simulink model "FuSimple"  (Simulink 5.0)
settings: Solver=ode23tb  StartTime=0.0  StopTime=inf  MaxStep=1/100000  MinStep=1/1000000000  RelTol=1e-6
undefined symbols (not defined in the file or in its folder): get, RFSSimple
libraries: simulink x7, commcontsrc2 x2, dspsnks4 x2
settings Model: LastModifiedBy=efst  SimulationMode=accelerator

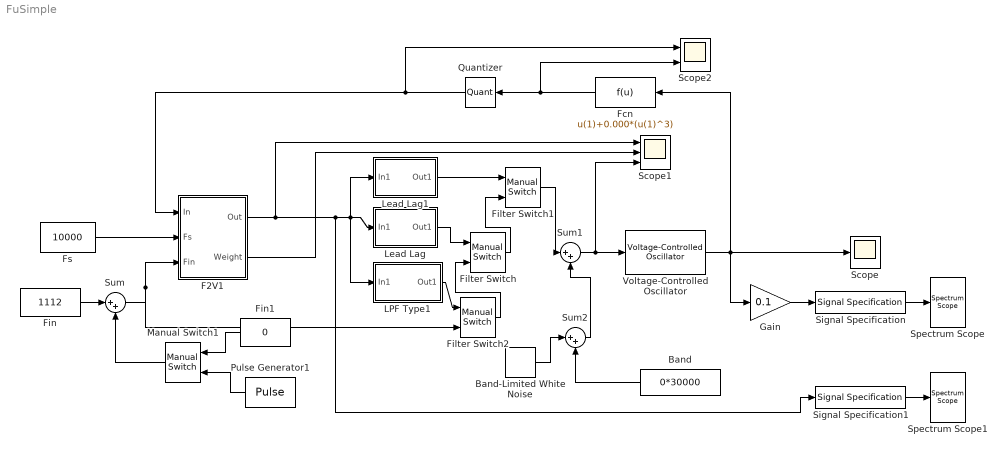
== system FuSimple ==
  Band : Constant  Orientation=left  Value=0*30000
  Band-Limited White Noise : simulink/Sources/Band-Limited White Noise  Cov=[0.0000]  Ts=1/10000  seed=[23341]
  F2V1 : Subsystem
  Fcn : Fcn  Orientation=left  Expr=u(1)+0.000*(u(1)^3)
  Filter Switch : simulink/Signal Routing/Manual Switch  sw=0  action=0
  Filter Switch1 : simulink/Signal Routing/Manual Switch  sw=0  action=0
  Filter Switch2 : simulink/Signal Routing/Manual Switch  sw=0  action=0
  Fin : Constant  Value=1112
  Fin1 : Constant  Orientation=left  Value=0
  Fs : Constant  Value=10000
  Gain : Gain  Gain=0.1  SaturateOnIntegerOverflow=on
  LPF Type1 : Subsystem  TreatAsAtomicUnit=on
  Lead Lag : Subsystem  TreatAsAtomicUnit=on
  Lead Lag1 : Subsystem  TreatAsAtomicUnit=on
  Manual Switch1 : simulink/Signal Routing/Manual Switch  Orientation=left  sw=1  action=0
  Pulse Generator1 : DiscretePulseGenerator  Orientation=left  PulseType=Time based  Amplitude=100  Period=1/90  PulseWidth=50
  Quantizer : Quantizer  Orientation=left  QuantizationInterval=2/(2^12)
  Scope : Scope
      settings: TimeRange=0.004496402877697842  YMin=-1  YMax=1
  Scope1 : Scope  NumInputPorts=3
      settings: TickLabels=on  TimeRange=0.1  YMin=-40~5.55112e-017~1110  YMax=90~1~1220
  Scope2 : Scope  NumInputPorts=2
      settings: TimeRange=0.003331112591605596  YMin=-1~-1  YMax=1~1  SaveName=ScopeData4
  Signal Specification : simulink/Signal Attributes/Signal Specification  D=1  Ts=1/10000  DataType=auto  OutDataType=sfix(16)  OutScaling=2^0
      settings: SignalType=auto  SamplingMode=sample-based
  Signal Specification1 : simulink/Signal Attributes/Signal Specification  D=1  Ts=1/10000  DataType=auto  OutDataType=sfix(16)  OutScaling=2^0
      settings: SignalType=auto  SamplingMode=sample-based
  Spectrum Scope : dspsnks4/Spectrum Scope  ScopeProperties=on  Domain=Frequency  HorizSpan=1  UseBuffer=on  BufferSize=2048  Overlap=64  inpFftLenInherit=on  FFTlength=2048  numAvg=2  DisplayProperties=off  AxisGrid=on  Memory=off  FrameNumber=on  AxisLegend=off  AxisZoom=off  OpenScopeAtSimStart=on  OpenScopeImmediately=off  FigPos=get(0,'defaultfigureposition')  AxisProperties=off  XUnits=Hertz  XRange=[0...Fs/2]  InheritXIncr=on  XIncr=1.0  XLabel=Samples  YUnits=dB  YLabel=Magnitude, dB  LineProperties=off
      settings: YMin=-164.609626558455  YMax=13.5929743373236
  Spectrum Scope1 : dspsnks4/Spectrum Scope  ScopeProperties=on  Domain=Frequency  HorizSpan=1  UseBuffer=on  BufferSize=2048  Overlap=64  inpFftLenInherit=on  FFTlength=2048  numAvg=2  DisplayProperties=off  AxisGrid=on  Memory=off  FrameNumber=on  AxisLegend=off  AxisZoom=off  OpenScopeAtSimStart=on  OpenScopeImmediately=off  FigPos=get(0,'defaultfigureposition')  AxisProperties=off  XUnits=Hertz  XRange=[0...Fs/2]  InheritXIncr=on  XIncr=1.0  XLabel=Samples  YUnits=dB  YLabel=Magnitude, dB  LineProperties=off  LineStyles=-  LineMarkers=.
      settings: YMin=-137.281906863743  YMax=1.3277218047623
  Sum : Sum  Inputs=|++  SaturateOnIntegerOverflow=on
  Sum1 : Sum  Inputs=|++  SaturateOnIntegerOverflow=on
  Sum2 : Sum  Inputs=|++  SaturateOnIntegerOverflow=on
  Voltage-Controlled Oscillator : commcontsrc2/Voltage-Controlled Oscillator  Ac=1  Fc=0  Kc=1  Ph=0
  wires:
  Signal Specification/1 -> Spectrum Scope/1
  F2V1/1(Out) -> Scope1/1, Lead Lag/1(In1), LPF Type1/1(In1), Lead Lag1/1(In1), Signal Specification1/1
  Fin/1 -> Sum/1
  Manual Switch1/1 -> Sum/2
  Pulse Generator1/1 -> Manual Switch1/2
  Fin1/1 -> Manual Switch1/1
  Sum1/1 -> Voltage-Controlled Oscillator/1, Scope1/3
  Gain/1 -> Signal Specification/1
  Lead Lag/1(Out1) -> Filter Switch/1
  Quantizer/1 -> F2V1/1(In), Scope2/1
  Fs/1 -> F2V1/2(Fs)
  Sum/1 -> F2V1/3(Fin), Filter Switch2/2
  Voltage-Controlled Oscillator/1 -> Scope/1, Gain/1, Fcn/1
  F2V1/2(Weight) -> Scope1/2
  Signal Specification1/1 -> Spectrum Scope1/1
  Fcn/1 -> Quantizer/1, Scope2/2
  Band-Limited White Noise/1 -> Sum2/1
  Sum2/1 -> Sum1/2
  Band/1 -> Sum2/2
  Filter Switch/1 -> Filter Switch1/2
  Lead Lag1/1(Out1) -> Filter Switch1/1
  Filter Switch1/1 -> Sum1/1
  Filter Switch2/1 -> Filter Switch/2
  LPF Type1/1(Out1) -> Filter Switch2/1

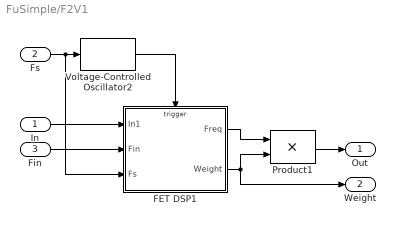
== system FuSimple/F2V1 ==
  In : Inport
  Fs : Inport  Port=2
  Fin : Inport  Port=3
  FET DSP1 : Subsystem  TreatAsAtomicUnit=on
  Product1 : Product  SaturateOnIntegerOverflow=on
  Voltage-Controlled Oscillator2 : commcontsrc2/Voltage-Controlled Oscillator  Ac=1  Fc=0  Kc=1  Ph=0
  Out : Outport
  Weight : Outport  Port=2
  wires:
  Fs/1 -> FET DSP1/3(Fs), Voltage-Controlled Oscillator2/1
  Product1/1 -> Out/1
  Fin/1 -> FET DSP1/2(Fin)
  In/1 -> FET DSP1/1(In1)
  FET DSP1/2(Weight) -> Weight/1, Product1/2
  FET DSP1/1(Freq) -> Product1/1
  Voltage-Controlled Oscillator2/1 -> FET DSP1/Trigger

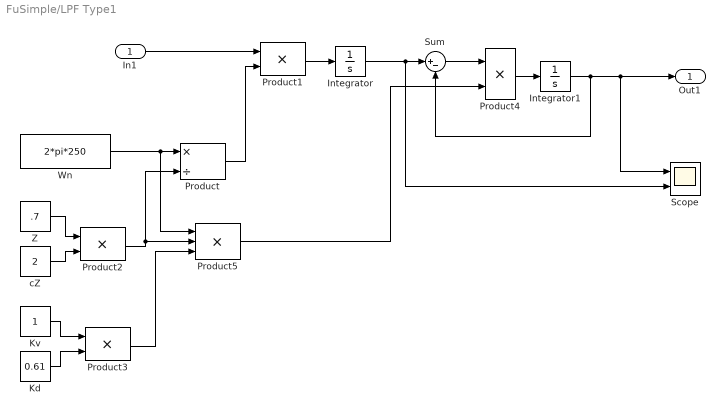
== system FuSimple/LPF Type1 ==
  In1 : Inport
  Integrator : Integrator  InitialCondition=2500  LimitOutput=on  UpperSaturationLimit=5000  LowerSaturationLimit=10
  Integrator1 : Integrator  InitialCondition=100  LimitOutput=on  UpperSaturationLimit=5000  LowerSaturationLimit=10
  Kd : Constant  Value=0.61
  Kv : Constant
  Product : Product  Inputs=*/  ShowAdditionalParam=on  RndMeth=Nearest  SaturateOnIntegerOverflow=on
  Product1 : Product  SaturateOnIntegerOverflow=on
  Product2 : Product  SaturateOnIntegerOverflow=on
  Product3 : Product  SaturateOnIntegerOverflow=on
  Product4 : Product  Inputs=**  SaturateOnIntegerOverflow=on
  Product5 : Product  Inputs=***  ShowAdditionalParam=on  RndMeth=Nearest  SaturateOnIntegerOverflow=on
  Scope : Scope  NumInputPorts=2
      settings: TimeRange=0.01  YMin=748.5~748  YMax=751~753  SaveName=ScopeData2
  Sum : Sum  Inputs=|+-  SaturateOnIntegerOverflow=on
  Wn : Constant  Value=2*pi*250
  Z : Constant  Value=.7
  cZ : Constant  Value=2
  Out1 : Outport
  wires:
  Product/1 -> Product1/2
  Z/1 -> Product2/1
  cZ/1 -> Product2/2
  Kv/1 -> Product3/1
  Kd/1 -> Product3/2
  Wn/1 -> Product/1, Product5/1
  Product1/1 -> Integrator/1
  Integrator/1 -> Sum/1, Scope/2
  In1/1 -> Product1/1
  Integrator1/1 -> Sum/2, Out1/1, Scope/1
  Sum/1 -> Product4/1
  Product4/1 -> Integrator1/1
  Product2/1 -> Product/2, Product5/2
  Product3/1 -> Product5/3
  Product5/1 -> Product4/2

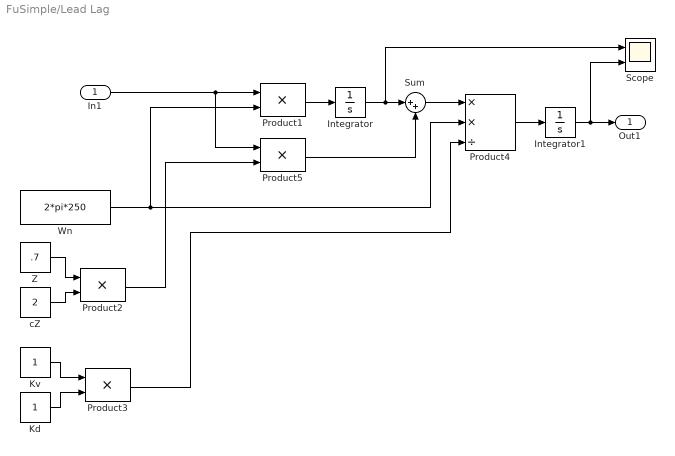
== system FuSimple/Lead Lag ==
  In1 : Inport
  Integrator : Integrator  UpperSaturationLimit=10  LowerSaturationLimit=-10  ZeroCross=off
  Integrator1 : Integrator  InitialCondition=1000  LimitOutput=on  UpperSaturationLimit=5000  LowerSaturationLimit=10
  Kd : Constant
  Kv : Constant
  Product{1..3,5} (4 alike) : Product  SaturateOnIntegerOverflow=on
  Product4 : Product  Inputs=**/  SaturateOnIntegerOverflow=on
  Scope : Scope  NumInputPorts=2
      settings: TimeRange=0.02  YMin=-10~490  YMax=7.5~515  SaveName=ScopeData3
  Sum : Sum  Inputs=|++  SaturateOnIntegerOverflow=on
  Wn : Constant  Value=2*pi*250
  Z : Constant  Value=.7
  cZ : Constant  Value=2
  Out1 : Outport
  wires:
  Z/1 -> Product2/1
  cZ/1 -> Product2/2
  Kv/1 -> Product3/1
  Kd/1 -> Product3/2
  Wn/1 -> Product1/2, Product4/2
  Product1/1 -> Integrator/1
  In1/1 -> Product1/1, Product5/1
  Integrator/1 -> Sum/1, Scope/1
  Product2/1 -> Product5/2
  Product5/1 -> Sum/2
  Sum/1 -> Product4/1
  Product3/1 -> Product4/3
  Product4/1 -> Integrator1/1
  Integrator1/1 -> Out1/1, Scope/2

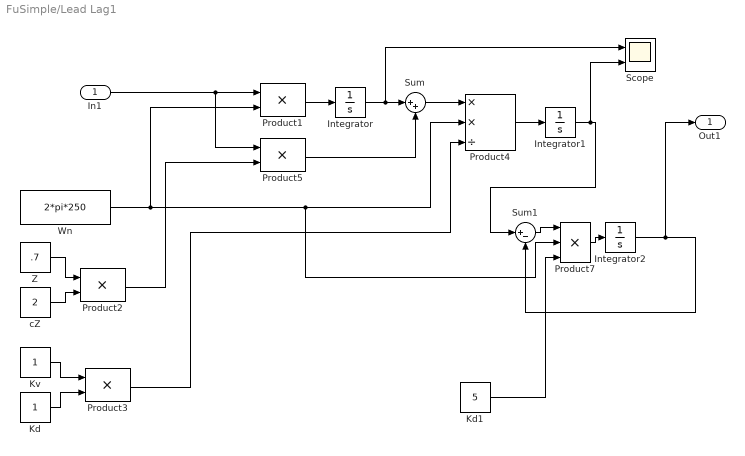
== system FuSimple/Lead Lag1 ==
  In1 : Inport
  Integrator : Integrator  UpperSaturationLimit=10  LowerSaturationLimit=-10  ZeroCross=off
  Integrator1 : Integrator  InitialCondition=1000  LimitOutput=on  UpperSaturationLimit=5000  LowerSaturationLimit=10
  Integrator2 : Integrator  UpperSaturationLimit=10  LowerSaturationLimit=-10  ZeroCross=off
  Kd : Constant
  Kd1 : Constant  Value=5
  Kv : Constant
  Product{1..3,5} (4 alike) : Product  SaturateOnIntegerOverflow=on
  Product4 : Product  Inputs=**/  SaturateOnIntegerOverflow=on
  Product7 : Product  Inputs=***  SaturateOnIntegerOverflow=on
  Scope : Scope  NumInputPorts=2
      settings: TimeRange=0.02  YMin=-10~490  YMax=7.5~515  SaveName=ScopeData3
  Sum : Sum  Inputs=|++  SaturateOnIntegerOverflow=on
  Sum1 : Sum  Inputs=|+-  SaturateOnIntegerOverflow=on
  Wn : Constant  Value=2*pi*250
  Z : Constant  Value=.7
  cZ : Constant  Value=2
  Out1 : Outport
  wires:
  Integrator1/1 -> Scope/2, Sum1/1
  Product4/1 -> Integrator1/1
  Product3/1 -> Product4/3
  Sum/1 -> Product4/1
  Product5/1 -> Sum/2
  Product2/1 -> Product5/2
  Integrator/1 -> Scope/1, Sum/1
  In1/1 -> Product5/1, Product1/1
  Product1/1 -> Integrator/1
  Wn/1 -> Product1/2, Product4/2, Product7/2
  Kd/1 -> Product3/2
  Kv/1 -> Product3/1
  cZ/1 -> Product2/2
  Z/1 -> Product2/1
  Integrator2/1 -> Out1/1, Sum1/2
  Sum1/1 -> Product7/1
  Product7/1 -> Integrator2/1
  Kd1/1 -> Product7/3

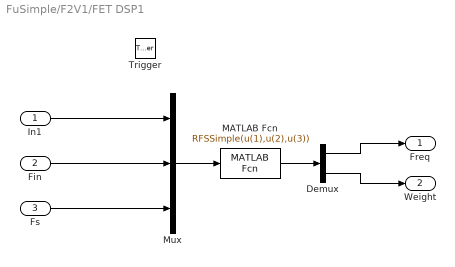
== system FuSimple/F2V1/FET DSP1 ==
  In1 : Inport
  Fin : Inport  Port=2
  Fs : Inport  Port=3
  Trigger : TriggerPort
  Demux : Demux  Outputs=2
  MATLAB Fcn : MATLABFcn  MATLABFcn=RFSSimple(u(1),u(2),u(3))  OutputDimensions=2  OutputSignalType=real
  Mux : Mux  Inputs=3
  Freq : Outport
  Weight : Outport  Port=2
  wires:
  Fin/1 -> Mux/2
  Mux/1 -> MATLAB Fcn/1
  In1/1 -> Mux/1
  Fs/1 -> Mux/3
  MATLAB Fcn/1 -> Demux/1
  Demux/1 -> Freq/1
  Demux/2 -> Weight/1
